simulink model "MutantsModel2"  (R2017b)
settings: Solver=ode3  StartTime=0.0  StopTime=inf  FixedStep=ts  RelTol=0.01  EnableMultiTasking=on
InitFcn:
  | ts=0.0005
  | %ts=100e-6;
StartFcn:
  | close all
StopFcn:
  | % Speed Torque Characterstic
  | 
  | 
  | %figure('Units','pixels', ...
  | %'Color',[1 1 1], ...
  | %'Name','Speed Torque Characterstic',...
  | %'NumberTitle','off',...
  | %'Position',[400 50 470 300], ...
  | %'ToolBar','none');
  | 
  | 
  | 
  | %plot(N_pi,Te_pi)
  | %title('Speed Torque Characterstic')
  | %xlabel('Speed [ RPM ]')
  | %ylabel('Electromagnetic Te_pi [ Nm ] ')
  | %grid on
  | %clear p4 p7 param5 param6 param8 parametres visible voltage
  | 
  | 
  | %clc
values from neighbouring files (symbols this model uses):
  TestOrder = [i]    [ExecuteTestSuite.m]    (also in mutants.m)
undefined symbols (not defined in the file or in its folder): emergency_button2, emergency_buttons, tc_simul, tc_size, temperature, trans1, trans2, trans3, trans4
libraries: simulink x44, powerlib_extras x11
(part 5 of 5)

== system MutantsModel2/mutant7/1 HP , 220 V Induction Motor/Measurements ==
  I_s : Inport
  I_r : Inport  Port=2
  I_ds : Inport  Port=3
  I_dr : Inport  Port=4
  I_qs : Inport  Port=5
  I_qr : Inport  Port=6
  Te : Inport  Port=7
  N : Inport  Port=8
  Bus Creator : BusCreator  Inputs=5
  Bus Creator1 : BusCreator  Inputs=5
  Bus Creator2 : BusCreator  Inputs=2
  Bus Creator3 : BusCreator  Inputs=3
  Demux : Demux  Outputs=3
  Demux1 : Demux  Outputs=3
  m : Outport
  wires:
  Bus Creator3/1 -> m/1
  Bus Creator2/1 -> Bus Creator3/3  "Mechanical"
  Bus Creator1/1 -> Bus Creator3/2  "Rotor Measurement"
  Bus Creator/1 -> Bus Creator3/1  "Stator Measurement"
  N/1 -> Bus Creator2/2  "Rotor Speed in (rpm)"
  Te/1 -> Bus Creator2/1  "Electromagnetic Torque (N*m)"
  I_qr/1 -> Bus Creator1/5  "Rotor Current i_qs (A)"
  I_dr/1 -> Bus Creator1/4  "Rotor Current i_ds (A)"
  Demux1/3 -> Bus Creator1/3  "Rotor Current i_sc (A)"
  Demux1/2 -> Bus Creator1/2  "Rotor Current i_sb (A)"
  Demux1/1 -> Bus Creator1/1  "Rotor Current i_sa (A)"
  I_r/1 -> Demux1/1
  I_qs/1 -> Bus Creator/5  "Stator Current i_qs (A)"
  I_ds/1 -> Bus Creator/4  "Stator Current i_ds (A)"
  Demux/3 -> Bus Creator/3  "Stator Current i_sc (A)"
  Demux/2 -> Bus Creator/2  "Stator Current i_sb (A)"
  Demux/1 -> Bus Creator/1  "Stator Current i_sa (A)"
  I_s/1 -> Demux/1

== system MutantsModel2/mutant7/1 HP , 220 V Induction Motor/Mechanical ==
  shi_ds : Inport
  shi_qs : Inport  Port=2
  i_ds : Inport  Port=3
  i_qs : Inport  Port=4
  tau : Inport  Port=5
  " " : Gain  Gain=P/2  SaturateOnIntegerOverflow=on  OutDataTypeStr=Inherit: Same as input  ParamDataTypeStr=Inherit: Same as input
  "  " : Gain  Gain=3*P/4  SaturateOnIntegerOverflow=on  OutDataTypeStr=Inherit: Same as input  ParamDataTypeStr=Inherit: Same as input
  1/J : Gain  Gain=1/J  SaturateOnIntegerOverflow=on  OutDataTypeStr=Inherit: Same as input  ParamDataTypeStr=Inherit: Same as input
  Integratorw : Integrator
  Product1 : Product
  Product2 : Product
  Sum : Sum  Inputs=+|-
  Sum5 : Sum  Inputs=+-  SaturateOnIntegerOverflow=on  InputSameDT=on  OutDataTypeStr=Inherit: Same as first input
  Te : Outport
  omegaR : Outport  Port=2
  we : Outport  Port=3
  wires:
  " "/1 -> we/1
  Integratorw/1 -> omegaR/1, " "/1
  1/J/1 -> Integratorw/1
  Sum5/1 -> 1/J/1
  tau/1 -> Sum5/2
  "  "/1 -> Sum5/1, Te/1
  Sum/1 -> "  "/1
  Product2/1 -> Sum/1
  Product1/1 -> Sum/2
  i_ds/1 -> Product1/2
  shi_qs/1 -> Product1/1
  i_qs/1 -> Product2/2
  shi_ds/1 -> Product2/1

== system MutantsModel2/mutant7/1 HP , 220 V Induction Motor/abc to dq ==
  Va : Inport
  Vb : Inport  Port=2
  Vc : Inport  Port=3
  "            " : Terminator
  Demux : Demux  Outputs=3
  Mux : Mux  Inputs=3
  abc2dq : Gain  Gain=[2/3 -1/3 -1/3; 0 sqrt(3)/3 -sqrt(3)/3; 1/3 1/3 1/3]  Multiplication=Matrix(K*u)  SaturateOnIntegerOverflow=on  OutDataTypeStr=Inherit: Same as input  ParamDataTypeStr=Inherit: Same as input
  V_ds : Outport
  V_qs : Outport  Port=2
  wires:
  Mux/1 -> abc2dq/1
  abc2dq/1 -> Demux/1
  Demux/2 -> V_qs/1
  Demux/1 -> V_ds/1
  Va/1 -> Mux/1
  Vb/1 -> Mux/2
  Vc/1 -> Mux/3
  Demux/3 -> "            "/1

== system MutantsModel2/mutant7/1 HP , 220 V Induction Motor/d_block ==
  shi_ds : Inport
  shi_dr : Inport  Port=2
  1/(Lr-((Lm*Lm)/Ls)) : Gain  Gain=1/(Lr-((Lm*Lm)/Ls))  SaturateOnIntegerOverflow=on  OutDataTypeStr=Inherit: Same as input  ParamDataTypeStr=Inherit: Same as input
  1/(Ls-((Lm*Lm)/Lr)) : Gain  Gain=1/(Ls-((Lm*Lm)/Lr))  SaturateOnIntegerOverflow=on  OutDataTypeStr=Inherit: Same as input  ParamDataTypeStr=Inherit: Same as input
  Lm/Lr : Gain  Gain=Lm/Lr
  Lm/Ls : Gain  Gain=Lm/Ls
  Sum : Sum  Inputs=|+-
  Sum1 : Sum  Inputs=-+|
  i_ds : Outport
  i_dr : Outport  Port=2
  wires:
  Sum1/1 -> 1/(Lr-((Lm*Lm)/Ls))/1
  Lm/Ls/1 -> Sum1/1
  Sum/1 -> 1/(Ls-((Lm*Lm)/Lr))/1
  Lm/Lr/1 -> Sum/2
  shi_dr/1 -> Sum1/2, Lm/Lr/1
  shi_ds/1 -> Lm/Ls/1, Sum/1
  1/(Lr-((Lm*Lm)/Ls))/1 -> i_dr/1
  1/(Ls-((Lm*Lm)/Lr))/1 -> i_ds/1

== system MutantsModel2/mutant7/1 HP , 220 V Induction Motor/dq to abc ==
  I_d : Inport
  I_q : Inport  Port=2
  Demux : Demux  Outputs=3
  Gain : Gain  Gain=2/3  SaturateOnIntegerOverflow=on  OutDataTypeStr=Inherit: Same as input  ParamDataTypeStr=Inherit: Same as input
  Matrix Gain : Gain  Gain=[1 0;-0.5 -sqrt(3)/2;-0.5 sqrt(3)/2]  Multiplication=Matrix(K*u)  SaturateOnIntegerOverflow=on  OutDataTypeStr=Inherit: Same as input  ParamDataTypeStr=Inherit: Same as input
  Mux : Mux  Inputs=2
  i_sa : Outport
  i_sb : Outport  Port=2
  i_sc : Outport  Port=3
  wires:
  Demux/1 -> i_sa/1
  Demux/3 -> i_sc/1
  I_q/1 -> Mux/2
  I_d/1 -> Mux/1
  Demux/2 -> i_sb/1
  Matrix Gain/1 -> Gain/1
  Gain/1 -> Demux/1
  Mux/1 -> Matrix Gain/1

== system MutantsModel2/mutant7/1 HP , 220 V Induction Motor/dq to abc  ==
  I_d : Inport
  I_q : Inport  Port=2
  Demux : Demux  Outputs=3
  Gain : Gain  Gain=2/3  SaturateOnIntegerOverflow=on  OutDataTypeStr=Inherit: Same as input  ParamDataTypeStr=Inherit: Same as input
  Matrix Gain : Gain  Gain=[1 0;-0.5 -sqrt(3)/2;-0.5 sqrt(3)/2]  Multiplication=Matrix(K*u)  SaturateOnIntegerOverflow=on  OutDataTypeStr=Inherit: Same as input  ParamDataTypeStr=Inherit: Same as input
  Mux : Mux  Inputs=2
  i_ra : Outport
  i_rb : Outport  Port=2
  i_rc : Outport  Port=3
  wires:
  Mux/1 -> Matrix Gain/1
  Gain/1 -> Demux/1
  Matrix Gain/1 -> Gain/1
  Demux/2 -> i_rb/1
  I_d/1 -> Mux/1
  I_q/1 -> Mux/2
  Demux/3 -> i_rc/1
  Demux/1 -> i_ra/1

== system MutantsModel2/mutant7/1 HP , 220 V Induction Motor/q_block ==
  shi_qs : Inport
  shi_qr : Inport  Port=2
  1/(Lr-((Lm*Lm)/Ls)) : Gain  Gain=1/(Lr-((Lm*Lm)/Ls))  SaturateOnIntegerOverflow=on  OutDataTypeStr=Inherit: Same as input  ParamDataTypeStr=Inherit: Same as input
  1/(Ls-((Lm*Lm)/Lr)) : Gain  Gain=1/(Ls-((Lm*Lm)/Lr))  SaturateOnIntegerOverflow=on  OutDataTypeStr=Inherit: Same as input  ParamDataTypeStr=Inherit: Same as input
  Lm/Lr : Gain  Gain=Lm/Lr
  Lm/Ls : Gain  Gain=Lm/Ls
  Sum : Sum  Inputs=|+-
  Sum1 : Sum  Inputs=-+|
  i_qs : Outport
  i_qr : Outport  Port=2
  wires:
  Sum1/1 -> 1/(Lr-((Lm*Lm)/Ls))/1
  Lm/Ls/1 -> Sum1/1
  Sum/1 -> 1/(Ls-((Lm*Lm)/Lr))/1
  Lm/Lr/1 -> Sum/2
  shi_qr/1 -> Lm/Lr/1, Sum1/2
  shi_qs/1 -> Lm/Ls/1, Sum/1
  1/(Lr-((Lm*Lm)/Ls))/1 -> i_qr/1
  1/(Ls-((Lm*Lm)/Lr))/1 -> i_qs/1

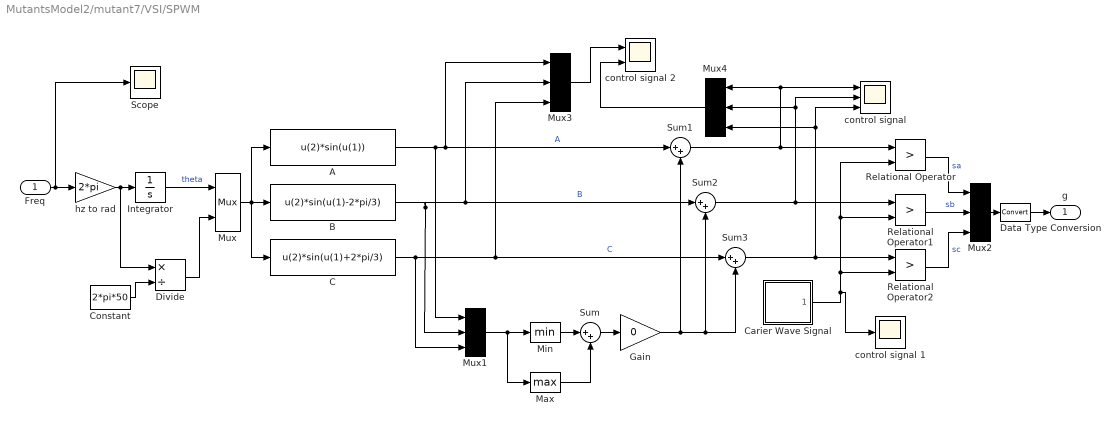
== system MutantsModel2/mutant7/VSI/SPWM ==
  Freq : Inport
  A : Fcn  Expr=u(2)*sin(u(1))
  B : Fcn  Expr=u(2)*sin(u(1)-2*pi/3)
  C : Fcn  Expr=u(2)*sin(u(1)+2*pi/3)
  Carier Wave Signal : Subsystem  mask(Carrier Wave Generator:){A=1, fc=500}
      mask prompts: A "Amplitude"; fc "Carrier Wave Frequency"
      mask Display: fprintf('Carrier\nWave')
  Constant : Constant  Value=2*pi*50
  Data Type Conversion : DataTypeConversion
  Divide : Product  Inputs=*/
  Gain : Gain  Gain=0
  Integrator : Integrator
  Max : MinMax  Function=max
  Min : MinMax
  Mux : Mux  Inputs=2
      settings: DisplayOption=signals
  Mux{1..4} (4 alike) : Mux  Inputs=3
      settings: DisplayOption=signals
  Relational Operator : RelationalOperator  Operator=>  OutDataTypeStr=boolean  RndMeth=Nearest
  Relational Operator1 : RelationalOperator  Operator=>  OutDataTypeStr=boolean  RndMeth=Nearest
  Relational Operator2 : RelationalOperator  Operator=>  OutDataTypeStr=boolean  RndMeth=Nearest
  Scope : Scope
  Sum{,1..3} (4 alike) : Sum  Inputs=|++
  "control signal " : Scope  NumInputPorts=3
  control signal 1 : Scope
  control signal 2 : Scope  NumInputPorts=2
  hz to rad : Gain  Gain=2*pi
  g : Outport
  wires:
  Mux4/1 -> control signal 2/2
  Mux3/1 -> control signal 2/1
  Constant/1 -> Divide/2
  Divide/1 -> Mux/2
  Gain/1 -> Sum1/2, Sum3/2, Sum2/2
  Freq/1 -> hz to rad/1, Scope/1
  C/1 -> Mux3/3, Sum3/1, Mux1/3  "C"
  Mux/1 -> C/1, A/1, B/1
  Integrator/1 -> Mux/1  "theta"
  A/1 -> Mux3/1, Sum1/1, Mux1/1  "A"
  hz to rad/1 -> Divide/1, Integrator/1
  B/1 -> Mux3/2, Sum2/1, Mux1/2  "B"
  Min/1 -> Sum/1
  Max/1 -> Sum/2
  Carier Wave Signal/1("Carier Wave ") -> control signal 1/1, Relational Operator2/2, Relational Operator1/2, Relational Operator/2
  Relational Operator2/1 -> Mux2/3  "sc"
  Relational Operator1/1 -> Mux2/2  "sb"
  Relational Operator/1 -> Mux2/1  "sa"
  Mux1/1 -> Max/1, Min/1
  Sum/1 -> Gain/1
  Sum1/1 -> Mux4/1, "control signal "/1, Relational Operator/1
  Sum2/1 -> Mux4/2, "control signal "/2, Relational Operator1/1
  Sum3/1 -> Mux4/3, "control signal "/3, Relational Operator2/1
  Mux2/1 -> Data Type Conversion/1
  Data Type Conversion/1 -> g/1

== system MutantsModel2/mutant8/1 HP , 220 V Induction Motor/Flux ==
  V_ds : Inport
  V_qs : Inport  Port=2
  I_ds : Inport  Port=3
  I_dr : Inport  Port=4
  I_qs : Inport  Port=5
  I_qr : Inport  Port=6
  we : Inport  Port=7
  Integrator{,1..3} (4 alike) : Integrator
  Product : Product
  Product1 : Product
  Rr : Gain  Gain=Rr
  "Rr " : Gain  Gain=Rr
  Rs : Gain  Gain=Rs
  "Rs " : Gain  Gain=Rs
  Sum : Sum  Inputs=+|-
  Sum1 : Sum  Inputs=+|-
  Sum2 : Sum  Inputs=|--
  Sum3 : Sum  Inputs=|+-
  shi_ds : Outport
  "shi_dr " : Outport  Port=2
  shi_qs : Outport  Port=3
  "shi_qr " : Outport  Port=4
  wires:
  I_ds/1 -> Rs/1
  V_ds/1 -> Sum/1
  Sum/1 -> Integrator/1
  I_qs/1 -> "Rs "/1
  V_qs/1 -> Sum1/1
  Sum1/1 -> Integrator1/1
  Integrator/1 -> shi_ds/1
  Integrator1/1 -> shi_qs/1
  Rs/1 -> Sum/2
  "Rs "/1 -> Sum1/2
  we/1 -> Product/2, Product1/1
  Integrator3/1 -> Product/1, "shi_qr "/1
  I_dr/1 -> Rr/1
  Rr/1 -> Sum2/2
  Product/1 -> Sum2/1
  Sum2/1 -> Integrator2/1
  Integrator2/1 -> Product1/2, "shi_dr "/1
  I_qr/1 -> "Rr "/1
  Product1/1 -> Sum3/1
  "Rr "/1 -> Sum3/2
  Sum3/1 -> Integrator3/1

== system MutantsModel2/mutant8/1 HP , 220 V Induction Motor/Measurements ==
  I_s : Inport
  I_r : Inport  Port=2
  I_ds : Inport  Port=3
  I_dr : Inport  Port=4
  I_qs : Inport  Port=5
  I_qr : Inport  Port=6
  Te : Inport  Port=7
  N : Inport  Port=8
  Bus Creator : BusCreator  Inputs=5
  Bus Creator1 : BusCreator  Inputs=5
  Bus Creator2 : BusCreator  Inputs=2
  Bus Creator3 : BusCreator  Inputs=3
  Demux : Demux  Outputs=3
  Demux1 : Demux  Outputs=3
  m : Outport
  wires:
  I_s/1 -> Demux/1
  Demux/1 -> Bus Creator/1  "Stator Current i_sa (A)"
  Demux/2 -> Bus Creator/2  "Stator Current i_sb (A)"
  Demux/3 -> Bus Creator/3  "Stator Current i_sc (A)"
  I_ds/1 -> Bus Creator/4  "Stator Current i_ds (A)"
  I_qs/1 -> Bus Creator/5  "Stator Current i_qs (A)"
  I_r/1 -> Demux1/1
  Demux1/1 -> Bus Creator1/1  "Rotor Current i_sa (A)"
  Demux1/2 -> Bus Creator1/2  "Rotor Current i_sb (A)"
  Demux1/3 -> Bus Creator1/3  "Rotor Current i_sc (A)"
  I_dr/1 -> Bus Creator1/4  "Rotor Current i_ds (A)"
  I_qr/1 -> Bus Creator1/5  "Rotor Current i_qs (A)"
  Te/1 -> Bus Creator2/1  "Electromagnetic Torque (N*m)"
  N/1 -> Bus Creator2/2  "Rotor Speed in (rpm)"
  Bus Creator/1 -> Bus Creator3/1  "Stator Measurement"
  Bus Creator1/1 -> Bus Creator3/2  "Rotor Measurement"
  Bus Creator2/1 -> Bus Creator3/3  "Mechanical"
  Bus Creator3/1 -> m/1

== system MutantsModel2/mutant8/1 HP , 220 V Induction Motor/Mechanical ==
  shi_ds : Inport
  shi_qs : Inport  Port=2
  i_ds : Inport  Port=3
  i_qs : Inport  Port=4
  tau : Inport  Port=5
  " " : Gain  Gain=P/2  SaturateOnIntegerOverflow=on  OutDataTypeStr=Inherit: Same as input  ParamDataTypeStr=Inherit: Same as input
  "  " : Gain  Gain=3*P/4  SaturateOnIntegerOverflow=on  OutDataTypeStr=Inherit: Same as input  ParamDataTypeStr=Inherit: Same as input
  1/J : Gain  Gain=1/J  SaturateOnIntegerOverflow=on  OutDataTypeStr=Inherit: Same as input  ParamDataTypeStr=Inherit: Same as input
  Integratorw : Integrator
  Product1 : Product
  Product2 : Product
  Sum : Sum  Inputs=+|-
  Sum5 : Sum  Inputs=+-  SaturateOnIntegerOverflow=on  InputSameDT=on  OutDataTypeStr=Inherit: Same as first input
  Te : Outport
  omegaR : Outport  Port=2
  we : Outport  Port=3
  wires:
  shi_ds/1 -> Product2/1
  i_qs/1 -> Product2/2
  shi_qs/1 -> Product1/1
  i_ds/1 -> Product1/2
  Product1/1 -> Sum/2
  Product2/1 -> Sum/1
  Sum/1 -> "  "/1
  "  "/1 -> Te/1, Sum5/1
  tau/1 -> Sum5/2
  Sum5/1 -> 1/J/1
  1/J/1 -> Integratorw/1
  Integratorw/1 -> " "/1, omegaR/1
  " "/1 -> we/1

== system MutantsModel2/mutant8/1 HP , 220 V Induction Motor/abc to dq ==
  Va : Inport
  Vb : Inport  Port=2
  Vc : Inport  Port=3
  "            " : Terminator
  Demux : Demux  Outputs=3
  Mux : Mux  Inputs=3
  abc2dq : Gain  Gain=[2/3 -1/3 -1/3; 0 sqrt(3)/3 -sqrt(3)/3; 1/3 1/3 1/3]  Multiplication=Matrix(K*u)  SaturateOnIntegerOverflow=on  OutDataTypeStr=Inherit: Same as input  ParamDataTypeStr=Inherit: Same as input
  V_ds : Outport
  V_qs : Outport  Port=2
  wires:
  Demux/3 -> "            "/1
  Vc/1 -> Mux/3
  Vb/1 -> Mux/2
  Va/1 -> Mux/1
  Demux/1 -> V_ds/1
  Demux/2 -> V_qs/1
  abc2dq/1 -> Demux/1
  Mux/1 -> abc2dq/1

== system MutantsModel2/mutant8/1 HP , 220 V Induction Motor/d_block ==
  shi_ds : Inport
  shi_dr : Inport  Port=2
  1/(Lr-((Lm*Lm)/Ls)) : Gain  Gain=1/(Lr-((Lm*Lm)/Ls))  SaturateOnIntegerOverflow=on  OutDataTypeStr=Inherit: Same as input  ParamDataTypeStr=Inherit: Same as input
  1/(Ls-((Lm*Lm)/Lr)) : Gain  Gain=1/(Ls-((Lm*Lm)/Lr))  SaturateOnIntegerOverflow=on  OutDataTypeStr=Inherit: Same as input  ParamDataTypeStr=Inherit: Same as input
  Lm/Lr : Gain  Gain=Lm/Lr
  Lm/Ls : Gain  Gain=Lm/Ls
  Sum : Sum  Inputs=|+-
  Sum1 : Sum  Inputs=-+|
  i_ds : Outport
  i_dr : Outport  Port=2
  wires:
  1/(Ls-((Lm*Lm)/Lr))/1 -> i_ds/1
  1/(Lr-((Lm*Lm)/Ls))/1 -> i_dr/1
  shi_ds/1 -> Sum/1, Lm/Ls/1
  shi_dr/1 -> Lm/Lr/1, Sum1/2
  Lm/Lr/1 -> Sum/2
  Sum/1 -> 1/(Ls-((Lm*Lm)/Lr))/1
  Lm/Ls/1 -> Sum1/1
  Sum1/1 -> 1/(Lr-((Lm*Lm)/Ls))/1

== system MutantsModel2/mutant8/1 HP , 220 V Induction Motor/dq to abc ==
  I_d : Inport
  I_q : Inport  Port=2
  Demux : Demux  Outputs=3
  Gain : Gain  Gain=2/3  SaturateOnIntegerOverflow=on  OutDataTypeStr=Inherit: Same as input  ParamDataTypeStr=Inherit: Same as input
  Matrix Gain : Gain  Gain=[1 0;-0.5 -sqrt(3)/2;-0.5 sqrt(3)/2]  Multiplication=Matrix(K*u)  SaturateOnIntegerOverflow=on  OutDataTypeStr=Inherit: Same as input  ParamDataTypeStr=Inherit: Same as input
  Mux : Mux  Inputs=2
  i_sa : Outport
  i_sb : Outport  Port=2
  i_sc : Outport  Port=3
  wires:
  Mux/1 -> Matrix Gain/1
  Gain/1 -> Demux/1
  Matrix Gain/1 -> Gain/1
  Demux/2 -> i_sb/1
  I_d/1 -> Mux/1
  I_q/1 -> Mux/2
  Demux/3 -> i_sc/1
  Demux/1 -> i_sa/1

== system MutantsModel2/mutant8/1 HP , 220 V Induction Motor/dq to abc  ==
  I_d : Inport
  I_q : Inport  Port=2
  Demux : Demux  Outputs=3
  Gain : Gain  Gain=2/3  SaturateOnIntegerOverflow=on  OutDataTypeStr=Inherit: Same as input  ParamDataTypeStr=Inherit: Same as input
  Matrix Gain : Gain  Gain=[1 0;-0.5 -sqrt(3)/2;-0.5 sqrt(3)/2]  Multiplication=Matrix(K*u)  SaturateOnIntegerOverflow=on  OutDataTypeStr=Inherit: Same as input  ParamDataTypeStr=Inherit: Same as input
  Mux : Mux  Inputs=2
  i_ra : Outport
  i_rb : Outport  Port=2
  i_rc : Outport  Port=3
  wires:
  Demux/1 -> i_ra/1
  Demux/3 -> i_rc/1
  I_q/1 -> Mux/2
  I_d/1 -> Mux/1
  Demux/2 -> i_rb/1
  Matrix Gain/1 -> Gain/1
  Gain/1 -> Demux/1
  Mux/1 -> Matrix Gain/1

== system MutantsModel2/mutant8/1 HP , 220 V Induction Motor/q_block ==
  shi_qs : Inport
  shi_qr : Inport  Port=2
  1/(Lr-((Lm*Lm)/Ls)) : Gain  Gain=1/(Lr-((Lm*Lm)/Ls))  SaturateOnIntegerOverflow=on  OutDataTypeStr=Inherit: Same as input  ParamDataTypeStr=Inherit: Same as input
  1/(Ls-((Lm*Lm)/Lr)) : Gain  Gain=1/(Ls-((Lm*Lm)/Lr))  SaturateOnIntegerOverflow=on  OutDataTypeStr=Inherit: Same as input  ParamDataTypeStr=Inherit: Same as input
  Lm/Lr : Gain  Gain=Lm/Lr
  Lm/Ls : Gain  Gain=Lm/Ls
  Sum : Sum  Inputs=|+-
  Sum1 : Sum  Inputs=-+|
  i_qs : Outport
  i_qr : Outport  Port=2
  wires:
  1/(Ls-((Lm*Lm)/Lr))/1 -> i_qs/1
  1/(Lr-((Lm*Lm)/Ls))/1 -> i_qr/1
  shi_qs/1 -> Sum/1, Lm/Ls/1
  shi_qr/1 -> Sum1/2, Lm/Lr/1
  Lm/Lr/1 -> Sum/2
  Sum/1 -> 1/(Ls-((Lm*Lm)/Lr))/1
  Lm/Ls/1 -> Sum1/1
  Sum1/1 -> 1/(Lr-((Lm*Lm)/Ls))/1

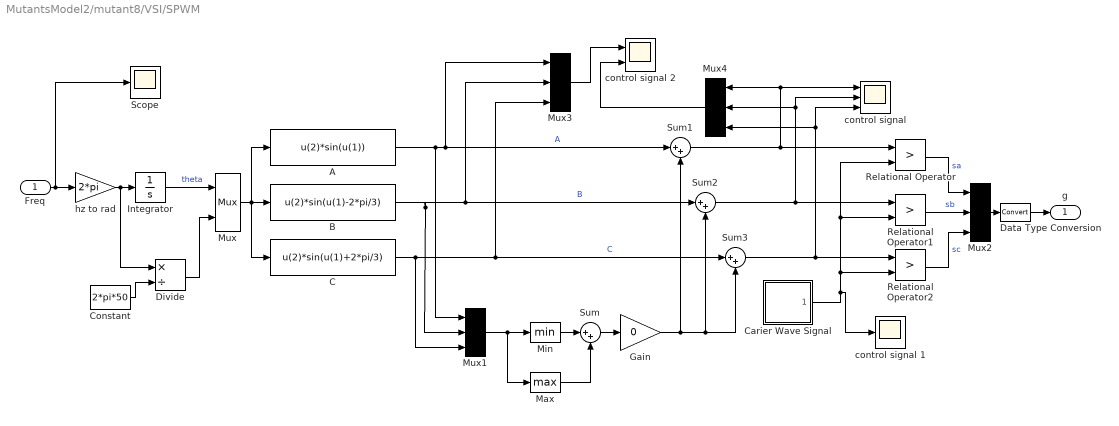
== system MutantsModel2/mutant8/VSI/SPWM ==
  Freq : Inport
  A : Fcn  Expr=u(2)*sin(u(1))
  B : Fcn  Expr=u(2)*sin(u(1)-2*pi/3)
  C : Fcn  Expr=u(2)*sin(u(1)+2*pi/3)
  Carier Wave Signal : Subsystem  mask(Carrier Wave Generator:){A=1, fc=500}
      mask prompts: A "Amplitude"; fc "Carrier Wave Frequency"
      mask Display: fprintf('Carrier\nWave')
  Constant : Constant  Value=2*pi*50
  Data Type Conversion : DataTypeConversion
  Divide : Product  Inputs=*/
  Gain : Gain  Gain=0
  Integrator : Integrator
  Max : MinMax  Function=max
  Min : MinMax
  Mux : Mux  Inputs=2
      settings: DisplayOption=signals
  Mux{1..4} (4 alike) : Mux  Inputs=3
      settings: DisplayOption=signals
  Relational Operator : RelationalOperator  Operator=>  OutDataTypeStr=boolean  RndMeth=Nearest
  Relational Operator1 : RelationalOperator  Operator=>  OutDataTypeStr=boolean  RndMeth=Nearest
  Relational Operator2 : RelationalOperator  Operator=>  OutDataTypeStr=boolean  RndMeth=Nearest
  Scope : Scope
  Sum{,1..3} (4 alike) : Sum  Inputs=|++
  "control signal " : Scope  NumInputPorts=3
  control signal 1 : Scope
  control signal 2 : Scope  NumInputPorts=2
  hz to rad : Gain  Gain=2*pi
  g : Outport
  wires:
  Data Type Conversion/1 -> g/1
  Mux2/1 -> Data Type Conversion/1
  Sum3/1 -> Relational Operator2/1, "control signal "/3, Mux4/3
  Sum2/1 -> Relational Operator1/1, "control signal "/2, Mux4/2
  Sum1/1 -> Relational Operator/1, "control signal "/1, Mux4/1
  Sum/1 -> Gain/1
  Mux1/1 -> Min/1, Max/1
  Relational Operator/1 -> Mux2/1  "sa"
  Relational Operator1/1 -> Mux2/2  "sb"
  Relational Operator2/1 -> Mux2/3  "sc"
  Carier Wave Signal/1("Carier Wave ") -> Relational Operator/2, Relational Operator1/2, Relational Operator2/2, control signal 1/1
  Max/1 -> Sum/2
  Min/1 -> Sum/1
  B/1 -> Mux1/2, Sum2/1, Mux3/2  "B"
  hz to rad/1 -> Integrator/1, Divide/1
  A/1 -> Mux1/1, Sum1/1, Mux3/1  "A"
  Integrator/1 -> Mux/1  "theta"
  Mux/1 -> B/1, A/1, C/1
  C/1 -> Mux1/3, Sum3/1, Mux3/3  "C"
  Freq/1 -> Scope/1, hz to rad/1
  Gain/1 -> Sum2/2, Sum3/2, Sum1/2
  Divide/1 -> Mux/2
  Constant/1 -> Divide/2
  Mux3/1 -> control signal 2/1
  Mux4/1 -> control signal 2/2

== system MutantsModel2/mutant9/1 HP , 220 V Induction Motor/Flux ==
  V_ds : Inport
  V_qs : Inport  Port=2
  I_ds : Inport  Port=3
  I_dr : Inport  Port=4
  I_qs : Inport  Port=5
  I_qr : Inport  Port=6
  we : Inport  Port=7
  Integrator{,1..3} (4 alike) : Integrator
  Product : Product
  Product1 : Product
  Rr : Gain  Gain=Rr
  "Rr " : Gain  Gain=Rr
  Rs : Gain  Gain=Rs
  "Rs " : Gain  Gain=Rs
  Sum : Sum  Inputs=+|-
  Sum1 : Sum  Inputs=+|-
  Sum2 : Sum  Inputs=|--
  Sum3 : Sum  Inputs=|+-
  shi_ds : Outport
  "shi_dr " : Outport  Port=2
  shi_qs : Outport  Port=3
  "shi_qr " : Outport  Port=4
  wires:
  Sum3/1 -> Integrator3/1
  "Rr "/1 -> Sum3/2
  Product1/1 -> Sum3/1
  I_qr/1 -> "Rr "/1
  Integrator2/1 -> "shi_dr "/1, Product1/2
  Sum2/1 -> Integrator2/1
  Product/1 -> Sum2/1
  Rr/1 -> Sum2/2
  I_dr/1 -> Rr/1
  Integrator3/1 -> "shi_qr "/1, Product/1
  we/1 -> Product1/1, Product/2
  "Rs "/1 -> Sum1/2
  Rs/1 -> Sum/2
  Integrator1/1 -> shi_qs/1
  Integrator/1 -> shi_ds/1
  Sum1/1 -> Integrator1/1
  V_qs/1 -> Sum1/1
  I_qs/1 -> "Rs "/1
  Sum/1 -> Integrator/1
  V_ds/1 -> Sum/1
  I_ds/1 -> Rs/1

== system MutantsModel2/mutant9/1 HP , 220 V Induction Motor/Measurements ==
  I_s : Inport
  I_r : Inport  Port=2
  I_ds : Inport  Port=3
  I_dr : Inport  Port=4
  I_qs : Inport  Port=5
  I_qr : Inport  Port=6
  Te : Inport  Port=7
  N : Inport  Port=8
  Bus Creator : BusCreator  Inputs=5
  Bus Creator1 : BusCreator  Inputs=5
  Bus Creator2 : BusCreator  Inputs=2
  Bus Creator3 : BusCreator  Inputs=3
  Demux : Demux  Outputs=3
  Demux1 : Demux  Outputs=3
  m : Outport
  wires:
  Bus Creator3/1 -> m/1
  Bus Creator2/1 -> Bus Creator3/3  "Mechanical"
  Bus Creator1/1 -> Bus Creator3/2  "Rotor Measurement"
  Bus Creator/1 -> Bus Creator3/1  "Stator Measurement"
  N/1 -> Bus Creator2/2  "Rotor Speed in (rpm)"
  Te/1 -> Bus Creator2/1  "Electromagnetic Torque (N*m)"
  I_qr/1 -> Bus Creator1/5  "Rotor Current i_qs (A)"
  I_dr/1 -> Bus Creator1/4  "Rotor Current i_ds (A)"
  Demux1/3 -> Bus Creator1/3  "Rotor Current i_sc (A)"
  Demux1/2 -> Bus Creator1/2  "Rotor Current i_sb (A)"
  Demux1/1 -> Bus Creator1/1  "Rotor Current i_sa (A)"
  I_r/1 -> Demux1/1
  I_qs/1 -> Bus Creator/5  "Stator Current i_qs (A)"
  I_ds/1 -> Bus Creator/4  "Stator Current i_ds (A)"
  Demux/3 -> Bus Creator/3  "Stator Current i_sc (A)"
  Demux/2 -> Bus Creator/2  "Stator Current i_sb (A)"
  Demux/1 -> Bus Creator/1  "Stator Current i_sa (A)"
  I_s/1 -> Demux/1

== system MutantsModel2/mutant9/1 HP , 220 V Induction Motor/Mechanical ==
  shi_ds : Inport
  shi_qs : Inport  Port=2
  i_ds : Inport  Port=3
  i_qs : Inport  Port=4
  tau : Inport  Port=5
  " " : Gain  Gain=P/2  SaturateOnIntegerOverflow=on  OutDataTypeStr=Inherit: Same as input  ParamDataTypeStr=Inherit: Same as input
  "  " : Gain  Gain=3*P/4  SaturateOnIntegerOverflow=on  OutDataTypeStr=Inherit: Same as input  ParamDataTypeStr=Inherit: Same as input
  1/J : Gain  Gain=1/J  SaturateOnIntegerOverflow=on  OutDataTypeStr=Inherit: Same as input  ParamDataTypeStr=Inherit: Same as input
  Integratorw : Integrator
  Product1 : Product
  Product2 : Product
  Sum : Sum  Inputs=+|-
  Sum5 : Sum  Inputs=+-  SaturateOnIntegerOverflow=on  InputSameDT=on  OutDataTypeStr=Inherit: Same as first input
  Te : Outport
  omegaR : Outport  Port=2
  we : Outport  Port=3
  wires:
  " "/1 -> we/1
  Integratorw/1 -> omegaR/1, " "/1
  1/J/1 -> Integratorw/1
  Sum5/1 -> 1/J/1
  tau/1 -> Sum5/2
  "  "/1 -> Sum5/1, Te/1
  Sum/1 -> "  "/1
  Product2/1 -> Sum/1
  Product1/1 -> Sum/2
  i_ds/1 -> Product1/2
  shi_qs/1 -> Product1/1
  i_qs/1 -> Product2/2
  shi_ds/1 -> Product2/1

== system MutantsModel2/mutant9/1 HP , 220 V Induction Motor/abc to dq ==
  Va : Inport
  Vb : Inport  Port=2
  Vc : Inport  Port=3
  "            " : Terminator
  Demux : Demux  Outputs=3
  Mux : Mux  Inputs=3
  abc2dq : Gain  Gain=[2/3 -1/3 -1/3; 0 sqrt(3)/3 -sqrt(3)/3; 1/3 1/3 1/3]  Multiplication=Matrix(K*u)  SaturateOnIntegerOverflow=on  OutDataTypeStr=Inherit: Same as input  ParamDataTypeStr=Inherit: Same as input
  V_ds : Outport
  V_qs : Outport  Port=2
  wires:
  Mux/1 -> abc2dq/1
  abc2dq/1 -> Demux/1
  Demux/2 -> V_qs/1
  Demux/1 -> V_ds/1
  Va/1 -> Mux/1
  Vb/1 -> Mux/2
  Vc/1 -> Mux/3
  Demux/3 -> "            "/1

== system MutantsModel2/mutant9/1 HP , 220 V Induction Motor/d_block ==
  shi_ds : Inport
  shi_dr : Inport  Port=2
  1/(Lr-((Lm*Lm)/Ls)) : Gain  Gain=1/(Lr-((Lm*Lm)/Ls))  SaturateOnIntegerOverflow=on  OutDataTypeStr=Inherit: Same as input  ParamDataTypeStr=Inherit: Same as input
  1/(Ls-((Lm*Lm)/Lr)) : Gain  Gain=1/(Ls-((Lm*Lm)/Lr))  SaturateOnIntegerOverflow=on  OutDataTypeStr=Inherit: Same as input  ParamDataTypeStr=Inherit: Same as input
  Lm/Lr : Gain  Gain=Lm/Lr
  Lm/Ls : Gain  Gain=Lm/Ls
  Sum : Sum  Inputs=|+-
  Sum1 : Sum  Inputs=-+|
  i_ds : Outport
  i_dr : Outport  Port=2
  wires:
  Sum1/1 -> 1/(Lr-((Lm*Lm)/Ls))/1
  Lm/Ls/1 -> Sum1/1
  Sum/1 -> 1/(Ls-((Lm*Lm)/Lr))/1
  Lm/Lr/1 -> Sum/2
  shi_dr/1 -> Sum1/2, Lm/Lr/1
  shi_ds/1 -> Lm/Ls/1, Sum/1
  1/(Lr-((Lm*Lm)/Ls))/1 -> i_dr/1
  1/(Ls-((Lm*Lm)/Lr))/1 -> i_ds/1

== system MutantsModel2/mutant9/1 HP , 220 V Induction Motor/dq to abc ==
  I_d : Inport
  I_q : Inport  Port=2
  Demux : Demux  Outputs=3
  Gain : Gain  Gain=2/3  SaturateOnIntegerOverflow=on  OutDataTypeStr=Inherit: Same as input  ParamDataTypeStr=Inherit: Same as input
  Matrix Gain : Gain  Gain=[1 0;-0.5 -sqrt(3)/2;-0.5 sqrt(3)/2]  Multiplication=Matrix(K*u)  SaturateOnIntegerOverflow=on  OutDataTypeStr=Inherit: Same as input  ParamDataTypeStr=Inherit: Same as input
  Mux : Mux  Inputs=2
  i_sa : Outport
  i_sb : Outport  Port=2
  i_sc : Outport  Port=3
  wires:
  Demux/1 -> i_sa/1
  Demux/3 -> i_sc/1
  I_q/1 -> Mux/2
  I_d/1 -> Mux/1
  Demux/2 -> i_sb/1
  Matrix Gain/1 -> Gain/1
  Gain/1 -> Demux/1
  Mux/1 -> Matrix Gain/1

== system MutantsModel2/mutant9/1 HP , 220 V Induction Motor/dq to abc  ==
  I_d : Inport
  I_q : Inport  Port=2
  Demux : Demux  Outputs=3
  Gain : Gain  Gain=2/3  SaturateOnIntegerOverflow=on  OutDataTypeStr=Inherit: Same as input  ParamDataTypeStr=Inherit: Same as input
  Matrix Gain : Gain  Gain=[1 0;-0.5 -sqrt(3)/2;-0.5 sqrt(3)/2]  Multiplication=Matrix(K*u)  SaturateOnIntegerOverflow=on  OutDataTypeStr=Inherit: Same as input  ParamDataTypeStr=Inherit: Same as input
  Mux : Mux  Inputs=2
  i_ra : Outport
  i_rb : Outport  Port=2
  i_rc : Outport  Port=3
  wires:
  Mux/1 -> Matrix Gain/1
  Gain/1 -> Demux/1
  Matrix Gain/1 -> Gain/1
  Demux/2 -> i_rb/1
  I_d/1 -> Mux/1
  I_q/1 -> Mux/2
  Demux/3 -> i_rc/1
  Demux/1 -> i_ra/1

== system MutantsModel2/mutant9/1 HP , 220 V Induction Motor/q_block ==
  shi_qs : Inport
  shi_qr : Inport  Port=2
  1/(Lr-((Lm*Lm)/Ls)) : Gain  Gain=1/(Lr-((Lm*Lm)/Ls))  SaturateOnIntegerOverflow=on  OutDataTypeStr=Inherit: Same as input  ParamDataTypeStr=Inherit: Same as input
  1/(Ls-((Lm*Lm)/Lr)) : Gain  Gain=1/(Ls-((Lm*Lm)/Lr))  SaturateOnIntegerOverflow=on  OutDataTypeStr=Inherit: Same as input  ParamDataTypeStr=Inherit: Same as input
  Lm/Lr : Gain  Gain=Lm/Lr
  Lm/Ls : Gain  Gain=Lm/Ls
  Sum : Sum  Inputs=|+-
  Sum1 : Sum  Inputs=-+|
  i_qs : Outport
  i_qr : Outport  Port=2
  wires:
  Sum1/1 -> 1/(Lr-((Lm*Lm)/Ls))/1
  Lm/Ls/1 -> Sum1/1
  Sum/1 -> 1/(Ls-((Lm*Lm)/Lr))/1
  Lm/Lr/1 -> Sum/2
  shi_qr/1 -> Lm/Lr/1, Sum1/2
  shi_qs/1 -> Lm/Ls/1, Sum/1
  1/(Lr-((Lm*Lm)/Ls))/1 -> i_qr/1
  1/(Ls-((Lm*Lm)/Lr))/1 -> i_qs/1

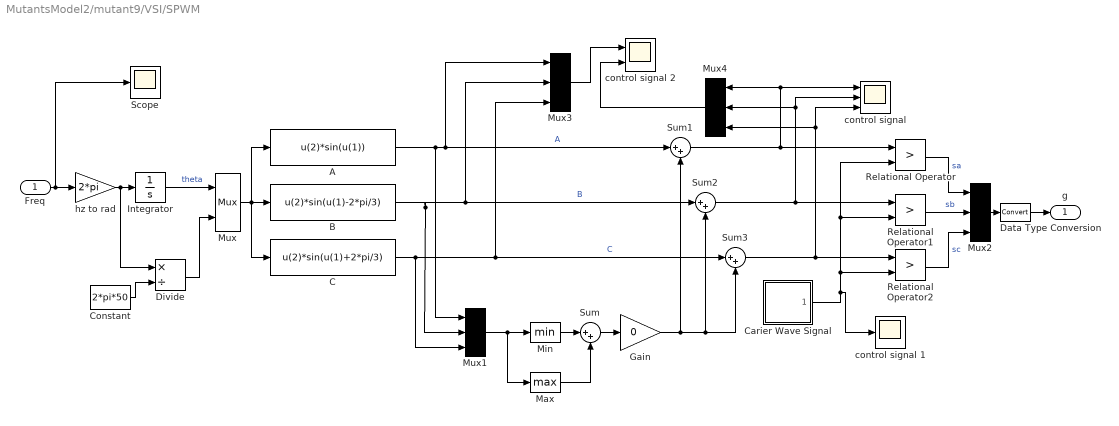
== system MutantsModel2/mutant9/VSI/SPWM ==
  Freq : Inport
  A : Fcn  Expr=u(2)*sin(u(1))
  B : Fcn  Expr=u(2)*sin(u(1)-2*pi/3)
  C : Fcn  Expr=u(2)*sin(u(1)+2*pi/3)
  Carier Wave Signal : Subsystem  mask(Carrier Wave Generator:){A=1, fc=500}
      mask prompts: A "Amplitude"; fc "Carrier Wave Frequency"
      mask Display: fprintf('Carrier\nWave')
  Constant : Constant  Value=2*pi*50
  Data Type Conversion : DataTypeConversion
  Divide : Product  Inputs=*/
  Gain : Gain  Gain=0
  Integrator : Integrator
  Max : MinMax  Function=max
  Min : MinMax
  Mux : Mux  Inputs=2
      settings: DisplayOption=signals
  Mux{1..4} (4 alike) : Mux  Inputs=3
      settings: DisplayOption=signals
  Relational Operator : RelationalOperator  Operator=>  OutDataTypeStr=boolean  RndMeth=Nearest
  Relational Operator1 : RelationalOperator  Operator=>  OutDataTypeStr=boolean  RndMeth=Nearest
  Relational Operator2 : RelationalOperator  Operator=>  OutDataTypeStr=boolean  RndMeth=Nearest
  Scope : Scope
  Sum{,1..3} (4 alike) : Sum  Inputs=|++
  "control signal " : Scope  NumInputPorts=3
  control signal 1 : Scope
  control signal 2 : Scope  NumInputPorts=2
  hz to rad : Gain  Gain=2*pi
  g : Outport
  wires:
  Mux4/1 -> control signal 2/2
  Mux3/1 -> control signal 2/1
  Constant/1 -> Divide/2
  Divide/1 -> Mux/2
  Gain/1 -> Sum1/2, Sum3/2, Sum2/2
  Freq/1 -> hz to rad/1, Scope/1
  C/1 -> Mux3/3, Sum3/1, Mux1/3  "C"
  Mux/1 -> C/1, A/1, B/1
  Integrator/1 -> Mux/1  "theta"
  A/1 -> Mux3/1, Sum1/1, Mux1/1  "A"
  hz to rad/1 -> Divide/1, Integrator/1
  B/1 -> Mux3/2, Sum2/1, Mux1/2  "B"
  Min/1 -> Sum/1
  Max/1 -> Sum/2
  Carier Wave Signal/1("Carier Wave ") -> control signal 1/1, Relational Operator2/2, Relational Operator1/2, Relational Operator/2
  Relational Operator2/1 -> Mux2/3  "sc"
  Relational Operator1/1 -> Mux2/2  "sb"
  Relational Operator/1 -> Mux2/1  "sa"
  Mux1/1 -> Max/1, Min/1
  Sum/1 -> Gain/1
  Sum1/1 -> Mux4/1, "control signal "/1, Relational Operator/1
  Sum2/1 -> Mux4/2, "control signal "/2, Relational Operator1/1
  Sum3/1 -> Mux4/3, "control signal "/3, Relational Operator2/1
  Mux2/1 -> Data Type Conversion/1
  Data Type Conversion/1 -> g/1

== system MutantsModel2/System/VSI/SPWM/Carier Wave Signal ==
  Carier Wave : simulink/Sources/Repeating Sequence  rep_seq_t=[0 0.25 0.5 0.75 1]./fc  rep_seq_y=[0 1 0 -1 0].*A
  "Carier Wave " : Outport
  wires:
  Carier Wave/1 -> "Carier Wave "/1  "0 delay"

== system MutantsModel2/mutant1/VSI/SPWM/Carier Wave Signal ==
  Carier Wave : simulink/Sources/Repeating Sequence  rep_seq_t=[0 0.25 0.5 0.75 1]./fc  rep_seq_y=[0 1 0 -1 0].*A
  "Carier Wave " : Outport
  wires:
  Carier Wave/1 -> "Carier Wave "/1  "0 delay"

== system MutantsModel2/mutant10/VSI/SPWM/Carier Wave Signal ==
  Carier Wave : simulink/Sources/Repeating Sequence  rep_seq_t=[0 0.25 0.5 0.75 1]./fc  rep_seq_y=[0 1 0 -1 0].*A
  "Carier Wave " : Outport
  wires:
  Carier Wave/1 -> "Carier Wave "/1  "0 delay"

== system MutantsModel2/mutant2/VSI/SPWM/Carier Wave Signal ==
  Carier Wave : simulink/Sources/Repeating Sequence  rep_seq_t=[0 0.25 0.5 0.75 1]./fc  rep_seq_y=[0 1 0 -1 0].*A
  "Carier Wave " : Outport
  wires:
  Carier Wave/1 -> "Carier Wave "/1  "0 delay"

== system MutantsModel2/mutant3/VSI/SPWM/Carier Wave Signal ==
  Carier Wave : simulink/Sources/Repeating Sequence  rep_seq_t=[0 0.25 0.5 0.75 1]./fc  rep_seq_y=[0 1 0 -1 0].*A
  "Carier Wave " : Outport
  wires:
  Carier Wave/1 -> "Carier Wave "/1  "0 delay"

== system MutantsModel2/mutant4/VSI/SPWM/Carier Wave Signal ==
  Carier Wave : simulink/Sources/Repeating Sequence  rep_seq_t=[0 0.25 0.5 0.75 1]./fc  rep_seq_y=[0 1 0 -1 0].*A
  "Carier Wave " : Outport
  wires:
  Carier Wave/1 -> "Carier Wave "/1  "0 delay"

== system MutantsModel2/mutant5/VSI/SPWM/Carier Wave Signal ==
  Carier Wave : simulink/Sources/Repeating Sequence  rep_seq_t=[0 0.25 0.5 0.75 1]./fc  rep_seq_y=[0 1 0 -1 0].*A
  "Carier Wave " : Outport
  wires:
  Carier Wave/1 -> "Carier Wave "/1  "0 delay"

== system MutantsModel2/mutant6/VSI/SPWM/Carier Wave Signal ==
  Carier Wave : simulink/Sources/Repeating Sequence  rep_seq_t=[0 0.25 0.5 0.75 1]./fc  rep_seq_y=[0 1 0 -1 0].*A
  "Carier Wave " : Outport
  wires:
  Carier Wave/1 -> "Carier Wave "/1  "0 delay"

== system MutantsModel2/mutant7/VSI/SPWM/Carier Wave Signal ==
  Carier Wave : simulink/Sources/Repeating Sequence  rep_seq_t=[0 0.25 0.5 0.75 1]./fc  rep_seq_y=[0 1 0 -1 0].*A
  "Carier Wave " : Outport
  wires:
  Carier Wave/1 -> "Carier Wave "/1  "0 delay"

== system MutantsModel2/mutant8/VSI/SPWM/Carier Wave Signal ==
  Carier Wave : simulink/Sources/Repeating Sequence  rep_seq_t=[0 0.25 0.5 0.75 1]./fc  rep_seq_y=[0 1 0 -1 0].*A
  "Carier Wave " : Outport
  wires:
  Carier Wave/1 -> "Carier Wave "/1  "0 delay"

== system MutantsModel2/mutant9/VSI/SPWM/Carier Wave Signal ==
  Carier Wave : simulink/Sources/Repeating Sequence  rep_seq_t=[0 0.25 0.5 0.75 1]./fc  rep_seq_y=[0 1 0 -1 0].*A
  "Carier Wave " : Outport
  wires:
  Carier Wave/1 -> "Carier Wave "/1  "0 delay"

== matlab function MutantsModel2/TestExecutor/MATLAB Function ==
  data: tc_simul input; port_1 output; test_case input; state input; port_2 output; port_3 output; port_4 output
function [port_1,port_2,port_3,port_4] = fcn(tc_simul, test_case, state)
%#codegen
    port_1 = tc_simul(test_case, 4*(state-1)+1);
    port_2 = tc_simul(test_case, 4*(state-1)+2);
    port_3 = tc_simul(test_case, 4*(state-1)+3);
    port_4 = tc_simul(test_case, 4*(state-1)+4);


end

== matlab function MutantsModel2/TestExecutor/MATLAB Function1 ==
  data: test_order input; tc_size input; trans1 input; trans2 input; trans3 input; trans4 input; v_engine input; temp input; test_order_id input; state_id input; test_case output; state output; test_order_id1 output; state_id1 output; simulation_stop output
function [test_case, state, test_order_id1, state_id1,simulation_stop] = fcn(test_order, tc_size, trans1,trans2, trans3, trans4, v_engine, temp,test_order_id,state_id)
%#codegen
    num_signals = 4;
    test_case = test_order(test_order_id);
    test_order_id1 = test_order_id;
    state = state_id;
    state_id1 = state;
    simulation_stop = false;
    
    if v_engine > trans1(test_case,state_id) && v_engine < trans2(test_case,state_id)
       if state_id<tc_size(test_case)/num_signals
          state = state_id+1;
          state_id1 = state;
       else
           if test_order_id1 < size(test_order,1)
               state = 1;
               state_id1 = state;
               test_order_id1 = test_order_id + 1;
           else
               simulation_stop = true;
               
           end
       end
    end

end
